simulink library "lab_6_task_2_simulink_library"  (R2025b)
settings: Solver=VariableStepAuto  StartTime=0.0  StopTime=10.0  RelTol=1e-3
libraries: matrix_library x1
settings Model: Creator=nicol  LastModifiedBy=nicol

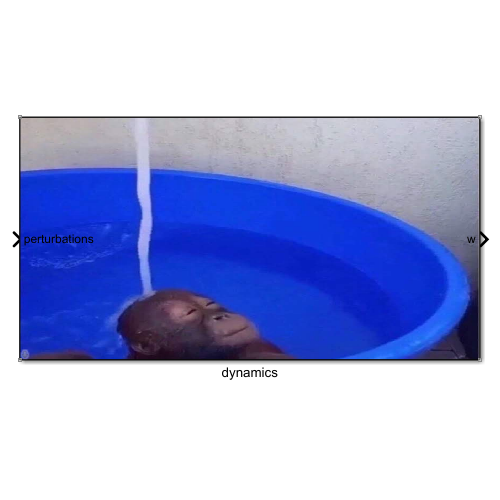
[thumbnail: Simulink's stored preview of the top-level diagram]
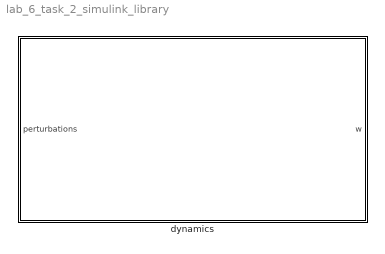
== system lab_6_task_2_simulink_library ==
  dynamics : Subsystem  mask{I=0, w0=0}
      mask prompts: I "Moment of Inertia Matrix [kg m^2]"; w0 "Initial Angular Velocity Matrix [rad s^-1]"
      mask DialogControl DescGroupVar Prompt: Rotation Dynamics w/ Gravity Gradient
      mask DialogControl DescTextVar Prompt: This is the block for rotation dynamics with gravity perturbation
      mask DialogControl ParameterGroupVar Prompt: Initial Condtions
      mask Display: image('little guy.jpeg');

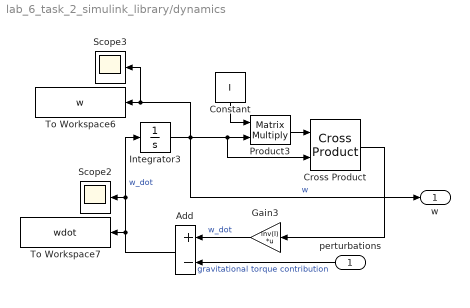
== system lab_6_task_2_simulink_library/dynamics ==
  perturbations : Inport
  Add : Sum  Inputs=+-
  Constant : Constant  Value=I
  Cross Product : matrix_library/Cross Product
  Gain3 : Gain  Gain=inv(I)  Multiplication=Matrix(K*u)
  Integrator3 : Integrator  InitialCondition=w0
  Product3 : Product  Multiplication=Matrix(*)
  Scope2 : Scope
      settings: ActiveDisplayYMinimum=-1  ActiveDisplayYMaximum=1  DataLoggingVariableName=ScopeData2
  Scope3 : Scope
      settings: ActiveDisplayYMinimum=-1  ActiveDisplayYMaximum=1  DataLoggingVariableName=ScopeData3
  To Workspace6 : ToWorkspace  VariableName=w  SaveFormat=Timeseries  SampleTime=-1
  To Workspace7 : ToWorkspace  VariableName=wdot  SaveFormat=Timeseries  SampleTime=-1
  w : Outport
  wires:
  Integrator3/1 -> w/1, Cross Product/2, Product3/2, To Workspace6/1, Scope3/1  "w"
  Cross Product/1 -> Gain3/1
  Add/1 -> Integrator3/1, Scope2/1, To Workspace7/1  "w_dot"
  Product3/1 -> Cross Product/1
  Constant/1 -> Product3/1
  Gain3/1 -> Add/1  "w_dot"
  perturbations/1 -> Add/2  "gravitational torque contribution"
